simulink model "Motor_Pos"  (R2017a)
settings: Solver=ode45  StartTime=0.0  StopTime=10.0  RelTol=1e-3
values from neighbouring files (symbols this model uses):
  b = 0.1    [setup_motor_position.m]
  J = 0.01    [setup_motor_position.m]
  K = 0.01    [setup_motor_position.m]
  L = 0.5    [setup_motor_position.m]
  R = 1.0    (= 1)    [setup_motor_position.m]
settings Model: Creator=sansh  LastModifiedBy=sansh

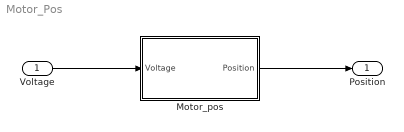
== system Motor_Pos ==
  Voltage : Inport
  Motor_pos : Subsystem
  Position : Outport
  wires:
  Voltage/1 -> Motor_pos/1(Voltage)
  Motor_pos/1(Position) -> Position/1

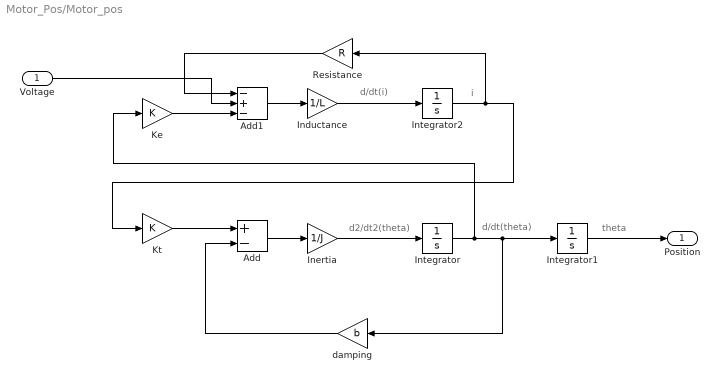
== system Motor_Pos/Motor_pos ==
  note: i
  note: d/dt(i)
  note: d2/dt2(theta)
  note: d/dt(theta)
  note: theta
  Voltage : Inport
  Add : Sum  Inputs=+-
  Add1 : Sum  Inputs=-+-
  Inductance : Gain  Gain=1/L
  Inertia : Gain  Gain=1/J
  Integrator : Integrator
  Integrator1 : Integrator
  Integrator2 : Integrator
  Ke : Gain  Gain=K
  Kt : Gain  Gain=K
  Resistance : Gain  Gain=R
  damping : Gain  Gain=b
  Position : Outport
  wires:
  Inertia/1 -> Integrator/1
  Inductance/1 -> Integrator2/1
  Integrator2/1 -> Resistance/1, Kt/1
  Integrator/1 -> Ke/1, damping/1, Integrator1/1
  Integrator1/1 -> Position/1
  Voltage/1 -> Add1/2
  Add/1 -> Inertia/1
  damping/1 -> Add/2
  Kt/1 -> Add/1
  Resistance/1 -> Add1/1
  Ke/1 -> Add1/3
  Add1/1 -> Inductance/1
